simulink model "PID_Parallel"  (R2024a)
settings: Solver=ode45  StartTime=0.0  StopTime=1  FixedStep=1e-2  RelTol=1e-4  AbsTol=1e-4
values from neighbouring files (symbols this model uses):
  Kp = 9.8    [ITAE_Plots_PT2_limitations Rechenbeispiel.m]
undefined symbols (not defined in the file or in its folder): Kd, Ki
settings Model: Creator=bhir  LastModifiedBy=Flo
settings SolverCC: AlgebraicLoopSolver=TrustRegion
settings DataIOCC: ReturnWorkspaceOutputs=off
settings DebuggingCC: UnconnectedInputMsg=warning  UnconnectedOutputMsg=warning  UnconnectedLineMsg=warning  ArithmeticOperatorsInVariantConditions=warning
settings SFSimCC: SimUseLocalCustomCode=off  CustomCodeUndefinedFunction=UseInterfaceOnly
settings RTWCC: RTWUseLocalCustomCode=off  GPUComputeCapability=3.5  DLArmComputeVersion=19.05
settings CodeAppCC: StateflowObjectComments=on

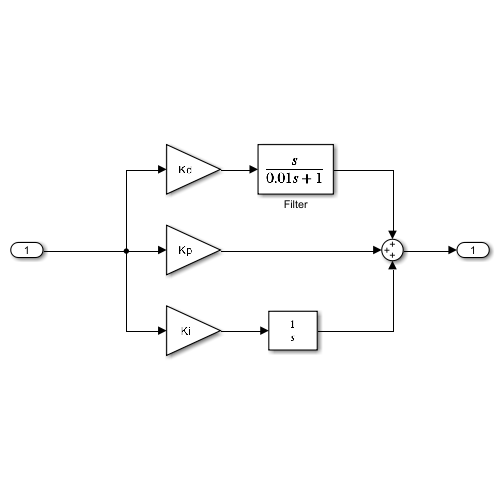
[thumbnail: Simulink's stored preview of the top-level diagram]
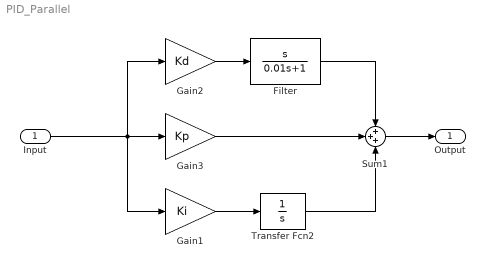
== system PID_Parallel ==
  Input : Inport
  Filter : TransferFcn  Numerator=[1 0]  Denominator=[0.01 1]
  Gain1 : Gain  Gain=Ki
  Gain2 : Gain  Gain=Kd
  Gain3 : Gain  Gain=Kp
  Sum1 : Sum  Inputs=+++
  Transfer Fcn2 : TransferFcn  Denominator=[1 0]
  Output : Outport
  wires:
  Gain1/1 -> Transfer Fcn2/1
  Input/1 -> Gain3/1, Gain1/1, Gain2/1
  Filter/1 -> Sum1/1
  Gain2/1 -> Filter/1
  Sum1/1 -> Output/1
  Transfer Fcn2/1 -> Sum1/3
  Gain3/1 -> Sum1/2
